simulink library "gsslib"  (R2015b)
settings: Solver=ode45  StartTime=0.0  StopTime=10.0  RelTol=1e-3
undefined symbols (not defined in the file or in its folder): ABCD, L
undefined symbols (not defined in the file): sys
libraries: cstblocks x1
settings Model: Creator=biannic  LastModifiedBy=croos
settings DataIOCC: SaveFormat=Array
settings OptimizationCC: ExpressionDepthLimit=2147483647
settings DebuggingCC: AlgebraicLoopMsg=none  UnderspecifiedInitializationDetection=Classic  MergeDetectMultiDrivingBlocksExec=none  SolverPrmCheckMsg=warning  StateNameClashWarn=warning
settings HardwareCC: ProdBitPerPointer=32  ProdLargestAtomicFloat=None  ProdIntDivRoundTo=Undefined  ProdEndianess=Unspecified  ProdWordSize=32  ProdHWDeviceType=32-bit Generic
settings GRTTargetCC: GeneratePreprocessorConditionals=Disable all
settings ConfigComp: CovModelRefEnable=Off

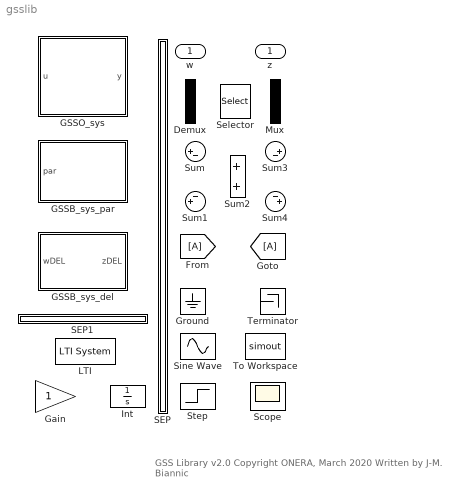
== system gsslib ==
  note: GSS Library v2.0
      | Copyright ONERA, March 2020
      | Written by  J-M. Biannic
  w : Inport
  Demux : Demux  Outputs=2
  GSSB_sys_del : Subsystem  mask(GSS LTI/NL DELTA BLOCK){sys=sys, del=del}
      mask prompts: sys "GSS object (gss)"; del "Non parametric Delta-block identifier (char)"
      mask help: This block enables to connect LTI or NL operators to a GSS object for simulation purpose.
      mask init:
      | initMASKGSSD
      mask Display:
      | color('red')
      | disp('{\bf GSS}', 'texmode', 'on');
      | color('black')
      | disp('\n\n\n DEL (LTI/NL)');
  GSSB_sys_par : Subsystem  mask(GSS PARAMETRIC BLOCK){sys=sys, par=par}
      mask prompts: sys "GSS object (gss)"; par "Parametric block identifier (char)"
      mask help: This block enables to assign time-varying or constant values from any source block. The user just needs to specify the name of the GSS object and that of the parameter.
      mask init:
      | initMASKGSSP
      mask Display:
      | color('red')
      | disp('\n\n')
      | disp('{\bf GSS}', 'texmode', 'on');
      | color('black')
      | disp('\n\n\n PARAMETER');
  GSSO_sys : Subsystem  mask(GSS OBJECT){sys=sys, x0=0}
      mask prompts: sys "GSS object"; x0 "Initial conditions (simulation only)"
      mask help:
      | y = Fu(M(s),DELTA)*u
      |
      | The LTI interconnection M(s) and the  block-diagonal structure and nature of the DELTA block are specified through the GSS object.
      |
      | This block is useful to compute interconnections of GSS objects  via Simulink with the routine slk2gss.
      |
      | It can also be used for simulation purpose. In that case, the values of DELTA are specified via additional objects (PAR or DEL) from the Library GSSLIB.
      mask init:
      | initMASKGSSO
      mask Display:
      | color('red')
      | disp('\n\n')
      | disp('{\bf GSS}', 'texmode', 'on');
      | color('black')
      | disp('\n\n\n OBJECT');
  Gain : Gain
  Ground : Ground
  Int : Integrator
  LTI : cstblocks/LTI System  sys=tf(1,[1 1])  IC=[]
  Mux : Mux  Inputs=2
  SEP : Subsystem
  SEP1 : Subsystem
  Scope : Scope
  Selector : Selector  InputPortWidth=2  IndexOptions=Index vector (dialog)  Indices=1  OutputSizes=1
  Sine Wave : Sin  SampleTime=0
  Step : Step  SampleTime=0
  Sum : Sum  Inputs=|+-
  Sum1 : Sum  Inputs=-+|
  Sum2 : Sum
  Sum3 : Sum  Inputs=|+-
  Sum4 : Sum  Inputs=-+|
  Terminator : Terminator
  To Workspace : ToWorkspace  VariableName=simout  SaveFormat=Timeseries  SampleTime=-1
  z : Outport

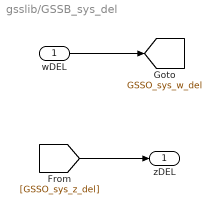
== system gsslib/GSSB_sys_del ==
  wDEL : Inport
  zDEL : Outport
  tag scope: GSSO_sys_w_del=global
  wires:
  wDEL/1 -> [GSSO_sys_w_del]
  [GSSO_sys_z_del] -> zDEL/1

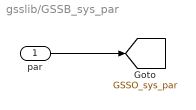
== system gsslib/GSSB_sys_par ==
  par : Inport
  tag scope: GSSO_sys_par=global
  wires:
  par/1 -> [GSSO_sys_par]

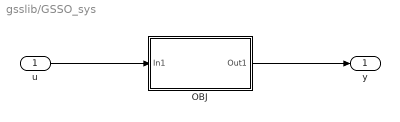
== system gsslib/GSSO_sys ==
  u : Inport
  OBJ : Subsystem
  y : Outport
  wires:
  u/1 -> OBJ/1(In1)
  OBJ/1(Out1) -> y/1

== system gsslib/SEP ==

== system gsslib/SEP1 ==

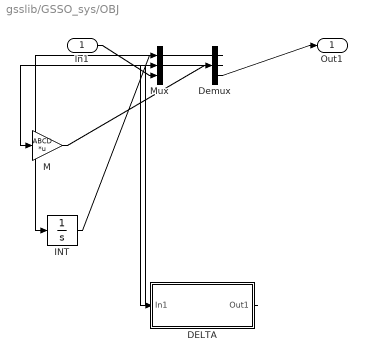
== system gsslib/GSSO_sys/OBJ ==
  In1 : Inport
  DELTA : Subsystem
  Demux : Demux  Outputs=dimDemux
  INT : Integrator
  M : Gain  Gain=ABCD  Multiplication=Matrix(K*u)
  Mux : Mux  Inputs=dimMux
  Out1 : Outport
  wires:
  Mux/1 -> M/1
  M/1 -> Demux/1
  Demux/1 -> INT/1
  INT/1 -> Mux/1
  Demux/2 -> DELTA/1(In1)
  DELTA/1(Out1) -> Mux/2
  In1/1 -> Mux/3
  Demux/3 -> Out1/1

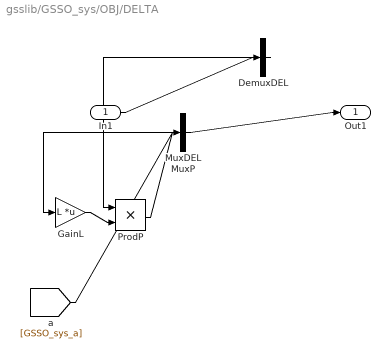
== system gsslib/GSSO_sys/OBJ/DELTA ==
  In1 : Inport
  DemuxDEL : Demux  Outputs=[ 2]
  GainL : Gain  Gain=L  Multiplication=Matrix(K*u)
  MuxDEL : Mux  Inputs=[ 2]
  MuxP : Mux  Inputs=1
  ProdP : Product  RndMeth=Zero
  Out1 : Outport
  wires:
  In1/1 -> DemuxDEL/1
  MuxDEL/1 -> Out1/1
  [GSSO_sys_a] -> MuxP/1
  MuxP/1 -> GainL/1
  DemuxDEL/1 -> ProdP/1
  GainL/1 -> ProdP/2
  ProdP/1 -> MuxDEL/1
